simulink model "tcp_client_test_slx"  (R2023a)
settings: Solver=ode5  StartTime=0.0  StopTime=2  FixedStep=0.001  RelTol=1e-3
libraries: simulink x1, sldrtlib x1
settings Model: Creator=chur  LastModifiedBy=chur
settings SolverCC: ConcurrentTasks=on  PositivePriorityOrder=on
settings OptimizationCC: BlockReduction=off  OptimizeBlockIOStorage=off
settings DebuggingCC: TasksWithSamePriorityMsg=none
settings HardwareCC: ProdBitPerLong=64  ProdHWDeviceType=Intel->x86-64 (Linux 64)
settings RTWCC: Description=Simulink Desktop Real-Time  SystemTargetFile=sldrt.tlc  TemplateMakefile=sldrt.tmf  Toolchain=Simulink Real-Time Toolchain  BuildConfiguration=Faster Runs  TargetLang=C++  RTWCompilerOptimization=on
settings CodeAppCC: MaxIdLength=95
settings SimulinkDesktopRealTimeCC: TargetLibSuffix=_sldrt.a  TargetPreCompLibLocation=D:\toolfile2\MATLAB R2023a\toolbox\sldrt\lib\win64  TargetLangStandard=C++03 (ISO)
settings ConfigComp: DVTestSuiteOptimization=Auto  DVDetectOutOfBounds=on  DVModelReferenceHarness=on  DVHarnessSource=Signal Editor

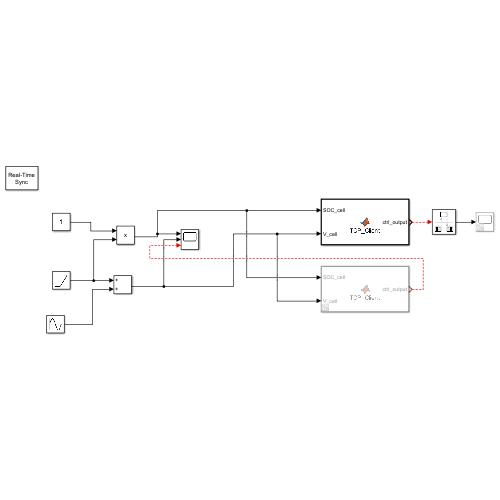
[thumbnail: Simulink's stored preview of the top-level diagram]
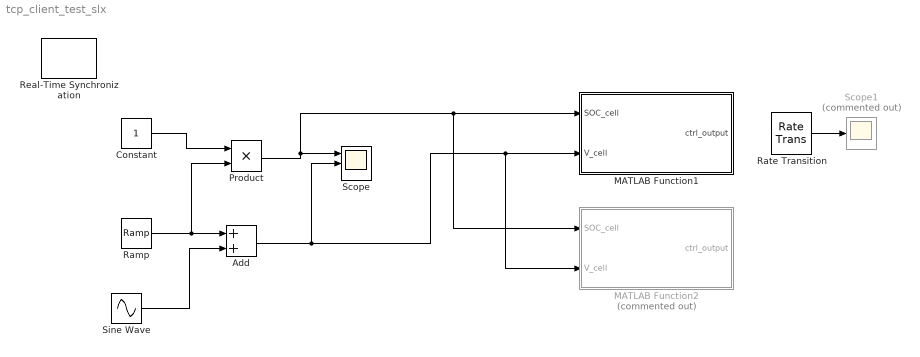
== system tcp_client_test_slx ==
  Add : Sum
  Constant : Constant
  MATLAB Function1 : MATLAB Function  TreatAsAtomicUnit=on
  MATLAB Function2 : MATLAB Function  Commented=on  TreatAsAtomicUnit=on
  Product : Product
  Ramp : simulink/Sources/Ramp  slope=1  start=0  InitialOutput=0
  Rate Transition : RateTransition  OutPortSampleTime=0.001
  Real-Time Synchronization : sldrtlib/Real-Time Synchronization  SampleTime=0.1  MaxMissedTicks=10  ShowMissedTicks=off  YieldWhenWaiting=off
  Scope : Scope  NumInputPorts=3
  Scope1 : Scope  Commented=on
  Sine Wave : Sin  SampleTime=0
  wires:
  Constant/1 -> Product/1
  Ramp/1 -> Add/1, Product/2
  Product/1 -> MATLAB Function2/1(SOC_cell), MATLAB Function1/1(SOC_cell), Scope/1
  Sine Wave/1 -> Add/2
  Add/1 -> Scope/2, MATLAB Function2/2(V_cell), MATLAB Function1/2(V_cell)
  ? -> Scope/3
  ? -> Rate Transition/1
  Rate Transition/1 -> Scope1/1

== matlab function tcp_client_test_slx/MATLAB Function1 ==
  data: SOC_cell input; V_cell input; ctrl_output output
%% connect to the TCP server (C++) in RevPi
function ctrl_output=TCP_Client(SOC_cell, V_cell)
    % coder.varsize('ctrl_output', [1 1]);  % Fixed size of 1
    % ctrl_output = double(0);             % Initialize with a double value

    tcp_client = tcpclient("192.168.137.2", 8080);  % Use 'localhost' if both client and server are on the same machine
    
    disp(['SOC_cell data type: ', class(SOC_cell)]);
    disp(['V_cell data type: ', class(V_cell)]);
    % Send a message to the server
    % write(tcp_client, uint8('Hello from MATLAB'));
    % Format the data as a string
    % data_to_send = sprintf('SOC:%.2f,V:%.2f', SOC_cell, V_cell);
    
    
    data_to_send = typecast(single([SOC_cell, V_cell]), 'uint8');
    write(tcp_client, data_to_send);
    
    % Specify the fixed length of the expected data (e.g., 8 bytes for two floats)
    fixed_length = 8;

    % Read exactly 8 bytes (2 floats)
    data = read(tcp_client, fixed_length);

    % Convert the raw bytes to floats
    % still try to fix this
    % float_data = typecast(uint8(data), 'single');

    % Display the received data (optional)
    disp('Received data:');
    % disp(data); 

    data = data(:);  % Reshape into a column vector
    float_data = typecast(uint8(data), 'single');
    ctrl_output =  float_data(1)+float_data(2);
    ctrl_output = double(ctrl_output);
    disp(ctrl_output);
    disp(['ctrl_output data type: ', class(ctrl_output)]);

    % disp(['float_data data type: ', class(float_data)]);
    % disp(float_data(1),float_data(2));
    
    % ctrl_output = 1.5;


end




% function modbusClient(SOC_cell, V_cell)
%     persistent client
%     if isempty(client)
%         % Connect to Modbus server on RevPi
%         client = modbus('tcpip', '192.168.137.2', 502);
%     end
% 
%     % Write SOC_cell to holding register 1
%     write(client, 'holdingregs', 1, round(SOC_cell * 100)); 
% 
%     % Write V_cell to holding register 2
%     write(client, 'holdingregs', 2, round(V_cell * 1000));
% end

% function modbusClient(SOC_cell, V_cell)
%     persistent client
%     if isempty(client)
%         % Connect to Modbus server on RevPi
%         client = modbus('tcpip', '192.168.137.2', 502);
%         disp('Connected to Modbus server');
%     end
% 
%     % Write SOC_cell to holding register 1
%     write(client, 'holdingregs', 1, round(SOC_cell * 100));
%     disp(['Sent SOC_cell to server: ', num2str(round(SOC_cell * 100))]);
% 
%     % Write V_cell to holding register 2
%     write(client, 'holdingregs', 2, round(V_cell * 1000));
%     disp(['Sent V_cell to server: ', num2str(round(V_cell * 1000))]);
% 
%     % Read response from server (e.g., holding register 0 for confirmation signal)
%     try
%         response = read(client, 'holdingregs', 0, 1); % Read 1 register starting at 0
%         disp(['Received confirmation from server: ', num2str(response(1))]);
%     catch ME
%         disp(['Failed to read response from server: ', ME.message]);
%     end
% end

== matlab function tcp_client_test_slx/MATLAB Function2 ==
  data: SOC_cell input; V_cell input; ctrl_output output
%% connect to the TCP server (C++) in RevPi
function ctrl_output=TCP_Client(SOC_cell, V_cell)
    
    
    ctrl_output =  SOC_cell+V_cell;
    


end




% function modbusClient(SOC_cell, V_cell)
%     persistent client
%     if isempty(client)
%         % Connect to Modbus server on RevPi
%         client = modbus('tcpip', '192.168.137.2', 502);
%     end
% 
%     % Write SOC_cell to holding register 1
%     write(client, 'holdingregs', 1, round(SOC_cell * 100)); 
% 
%     % Write V_cell to holding register 2
%     write(client, 'holdingregs', 2, round(V_cell * 1000));
% end

% function modbusClient(SOC_cell, V_cell)
%     persistent client
%     if isempty(client)
%         % Connect to Modbus server on RevPi
%         client = modbus('tcpip', '192.168.137.2', 502);
%         disp('Connected to Modbus server');
%     end
% 
%     % Write SOC_cell to holding register 1
%     write(client, 'holdingregs', 1, round(SOC_cell * 100));
%     disp(['Sent SOC_cell to server: ', num2str(round(SOC_cell * 100))]);
% 
%     % Write V_cell to holding register 2
%     write(client, 'holdingregs', 2, round(V_cell * 1000));
%     disp(['Sent V_cell to server: ', num2str(round(V_cell * 1000))]);
% 
%     % Read response from server (e.g., holding register 0 for confirmation signal)
%     try
%         response = read(client, 'holdingregs', 0, 1); % Read 1 register starting at 0
%         disp(['Received confirmation from server: ', num2str(response(1))]);
%     catch ME
%         disp(['Failed to read response from server: ', ME.message]);
%     end
% end
